simulink model "untitled1"  (R2017b)
settings: Solver=VariableStepAuto  StartTime=0.0  StopTime=10.0  RelTol=1e-3
settings Model: Creator=yaozhong.zhang  LastModifiedBy=yaozhong.zhang

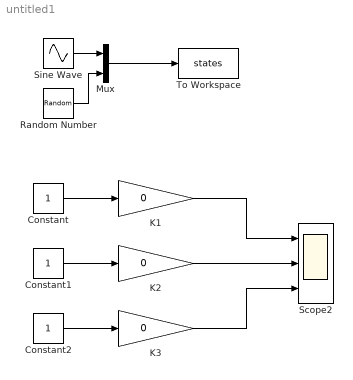
== system untitled1 ==
  Constant : Constant
  Constant1 : Constant
  Constant2 : Constant
  K1 : Gain  Gain=0
  K2 : Gain  Gain=0
  K3 : Gain  Gain=0
  Mux : Mux  Inputs=2
  Random Number : RandomNumber  SampleTime=0.1
  Scope2 : Scope  NumInputPorts=3
  Sine Wave : Sin  SampleTime=0
  To Workspace : ToWorkspace  VariableName=states  SaveFormat=Timeseries  SampleTime=-1
  wires:
  K3/1 -> Scope2/3
  Constant2/1 -> K3/1
  K2/1 -> Scope2/2
  Mux/1 -> To Workspace/1
  Constant/1 -> K1/1
  Sine Wave/1 -> Mux/1
  Constant1/1 -> K2/1
  Random Number/1 -> Mux/2
  K1/1 -> Scope2/1
